simulink model "Observador_controlador"  (R2015a)
settings: Solver=ode45  SolverMode=SingleTasking  StartTime=0.0  StopTime=10.0  RelTol=1e-3
undefined symbols (not defined in the file): Ts
settings Model: CovModelRefEnable=off  Creator=n221  LastModifiedBy=ARTURO
settings DataIOCC: SignalLoggingSaveFormat=ModelDataLogs
settings OptimizationCC: BlockReduction=off  BooleanDataType=off  ExpressionDepthLimit=2147483647
settings DebuggingCC: SaveWithParameterizedLinksMsg=none  UnderspecifiedInitializationDetection=Classic  MergeDetectMultiDrivingBlocksExec=none  SignalResolutionControl=TryResolveAllWithWarning  MultiTaskDSMMsg=warning  MultiTaskCondExecSysMsg=none  StateNameClashWarn=warning
settings HardwareCC: TargetUnknown=on

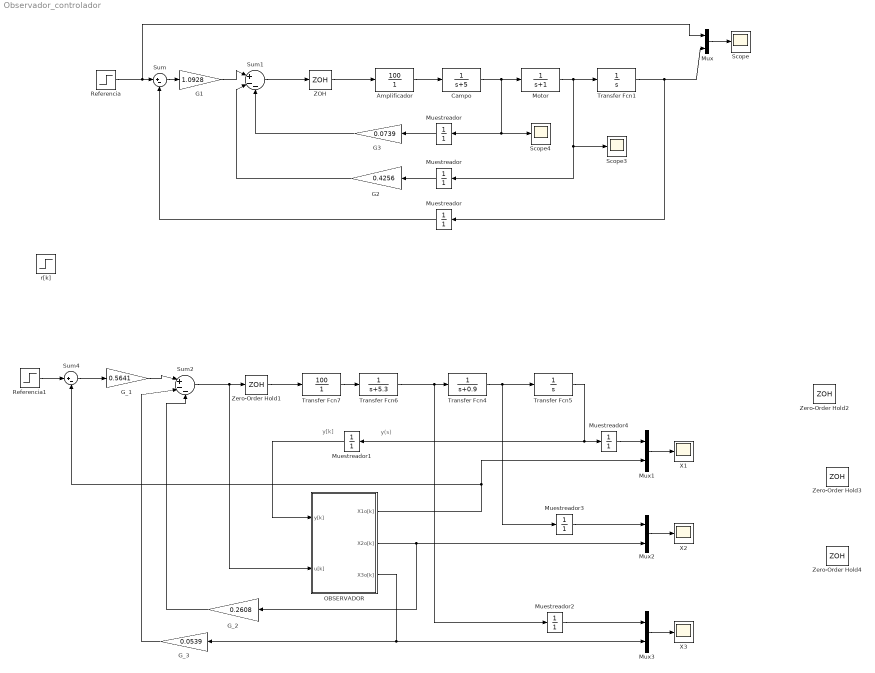
== system Observador_controlador ==
  note: y[k]
  note: y(s)
   Muestreador{,1..4} (5 alike) : DiscreteTransferFcn  Denominator=[1]  SampleTime=Ts
  Amplificador : TransferFcn  Numerator=[100]  Denominator=[1]
  Campo : TransferFcn  Denominator=[1 5]
  G1 : Gain  Gain=1.0928
  G2 : Gain  Gain=0.4256
  G3 : Gain  Gain=0.0739
  G_1 : Gain  Gain=0.5641
  G_2 : Gain  Gain=0.2608
  G_3 : Gain  Gain=0.0539
  Motor : TransferFcn  Denominator=[1 1]
  Muestreador : DiscreteTransferFcn  Denominator=[1]  SampleTime=Ts
  "Muestreador " : DiscreteTransferFcn  Denominator=[1]  SampleTime=Ts
  Mux{,1..3} (4 alike) : Mux  Inputs=2
  OBSERVADOR : Subsystem
  Referencia : Step  Time=0  SampleTime=Ts
  Referencia1 : Step  Time=0  SampleTime=Ts
  Scope : Scope
      settings: YMin=-0.13042  YMax=1.1738  SaveName=input_output
  Scope3 : Scope
      settings: YMin=-0.13042  YMax=1.1738  SaveName=input_output3
  Scope4 : Scope
      settings: YMin=-0.13042  YMax=1.1738  SaveName=input_output4
  Sum : Sum  Inputs=|+-
  Sum1 : Sum  Inputs=|+--
  Sum2 : Sum  Inputs=|+--
  Sum4 : Sum  Inputs=|+-
  Transfer Fcn1 : TransferFcn  Denominator=[1 0]
  Transfer Fcn4 : TransferFcn  Denominator=[1 0.9]
  Transfer Fcn5 : TransferFcn  Denominator=[1 0]
  Transfer Fcn6 : TransferFcn  Denominator=[1 5.3]
  Transfer Fcn7 : TransferFcn  Numerator=[100]  Denominator=[1]
  X1 : Scope
      settings: YMin=-0.13042  YMax=1.1738  SaveName=X1O
  X2 : Scope
      settings: YMin=-0.13042  YMax=1.1738  SaveName=X2O
  X3 : Scope
      settings: YMin=-0.13042  YMax=1.1738  SaveName=X3O
  ZOH : ZeroOrderHold  SampleTime=Ts
  Zero-Order Hold{1..4} (4 alike) : ZeroOrderHold  SampleTime=Ts
  r[k] : Step  Time=0  SampleTime=Ts
  wires:
  Motor/1 -> "Muestreador "/1, Scope3/1, Transfer Fcn1/1
  Campo/1 -> Muestreador/1, Scope4/1, Motor/1
  Amplificador/1 -> Campo/1
  ZOH/1 -> Amplificador/1
  Sum/1 -> G1/1
  Referencia/1 -> Sum/1, Mux/1
  G2/1 -> Sum1/2
  G1/1 -> Sum1/1
  Muestreador/1 -> G3/1
  "Muestreador "/1 -> G2/1
  Mux/1 -> Scope/1
  Transfer Fcn6/1 -> " Muestreador2"/1, Transfer Fcn4/1
  Transfer Fcn7/1 -> Transfer Fcn6/1
  Zero-Order Hold1/1 -> Transfer Fcn7/1
  " Muestreador"/1 -> Sum/2
  G3/1 -> Sum1/3
  Sum2/1 -> OBSERVADOR/2(u[k]), Zero-Order Hold1/1
  Referencia1/1 -> Sum4/1
  Sum4/1 -> G_1/1
  G_1/1 -> Sum2/1
  G_2/1 -> Sum2/3
  G_3/1 -> Sum2/2
  Mux1/1 -> X1/1
  OBSERVADOR/1(X1o[k]) -> Sum4/2, Mux1/2
  Transfer Fcn4/1 -> " Muestreador3"/1, Transfer Fcn5/1
  Mux2/1 -> X2/1
  OBSERVADOR/2(X2o[k]) -> Mux2/2, G_2/1
  Mux3/1 -> X3/1
  " Muestreador1"/1 -> OBSERVADOR/1(y[k])
  " Muestreador2"/1 -> Mux3/1
  " Muestreador3"/1 -> Mux2/1
  Transfer Fcn1/1 -> " Muestreador"/1, Mux/2
  Transfer Fcn5/1 -> " Muestreador1"/1, " Muestreador4"/1
  " Muestreador4"/1 -> Mux1/1
  Sum1/1 -> ZOH/1
  OBSERVADOR/3(X3o[k]) -> Mux3/2, G_3/1

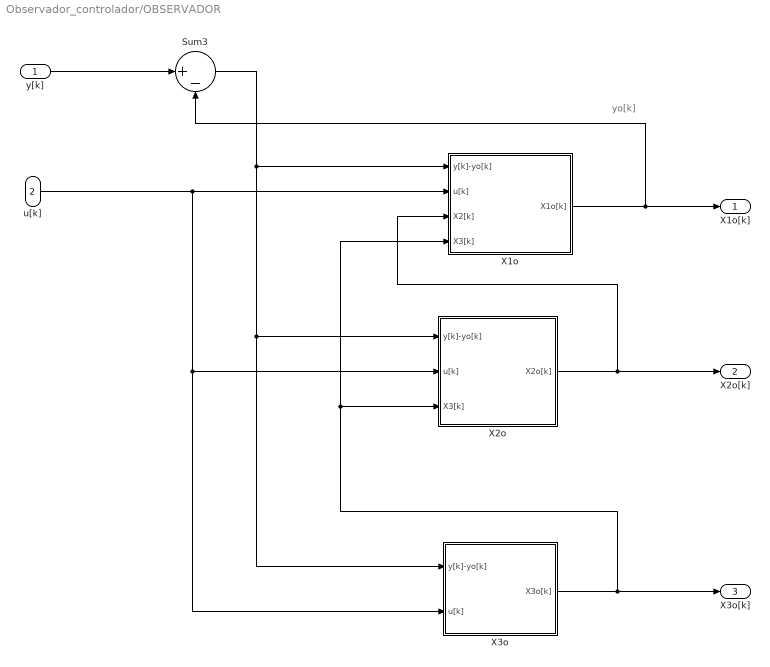
== system Observador_controlador/OBSERVADOR ==
  note: yo[k]
  y[k] : Inport
  u[k] : Inport  Port=2
  Sum3 : Sum  Inputs=|+-
  X1o : Subsystem
  X2o : Subsystem
  X3o : Subsystem
  X1o[k] : Outport
  X2o[k] : Outport  Port=2
  X3o[k] : Outport  Port=3
  wires:
  y[k]/1 -> Sum3/1
  Sum3/1 -> X3o/1(y[k]-yo[k]), X2o/1(y[k]-yo[k]), X1o/1(y[k]-yo[k])
  X2o/1(X2o[k]) -> X2o[k]/1, X1o/3(X2[k])
  u[k]/1 -> X3o/2(u[k]), X2o/2(u[k]), X1o/2(u[k])
  X3o/1(X3o[k]) -> X3o[k]/1, X2o/3(X3[k]), X1o/4(X3[k])
  X1o/1(X1o[k]) -> X1o[k]/1, Sum3/2

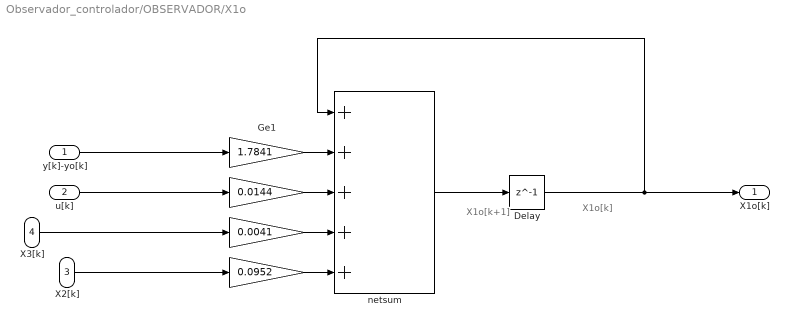
== system Observador_controlador/OBSERVADOR/X1o ==
  note: X1o[k]
  note: X1o[k+1]
  y[k]-yo[k] : Inport
  u[k] : Inport  Port=2
  X2[k] : Inport  Port=3
  X3[k] : Inport  Port=4
  " " : Gain  Gain=0.0144
  "   " : Gain  Gain=0.0952
  "    " : Gain  Gain=0.0041
  Delay : Delay  DelayLength=1  InitialCondition=0
  Ge1 : Gain  Gain=1.7841
  netsum : Sum  Inputs=5  SaturateOnIntegerOverflow=on  InputSameDT=on  OutDataTypeStr=Inherit: Same as first input
  X1o[k] : Outport
  wires:
  " "/1 -> netsum/3
  "    "/1 -> netsum/4
  "   "/1 -> netsum/5
  netsum/1 -> Delay/1
  Ge1/1 -> netsum/2
  Delay/1 -> netsum/1, X1o[k]/1
  X3[k]/1 -> "    "/1
  u[k]/1 -> " "/1
  X2[k]/1 -> "   "/1
  y[k]-yo[k]/1 -> Ge1/1

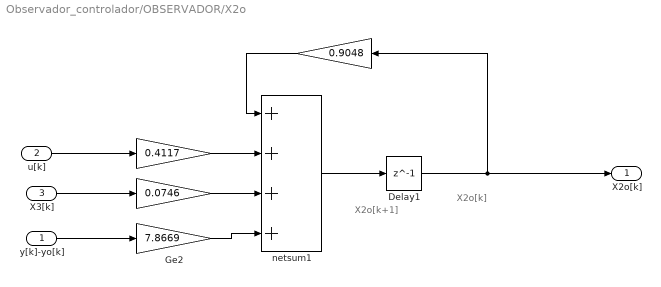
== system Observador_controlador/OBSERVADOR/X2o ==
  note: X2o[k]
  note: X2o[k+1]
  y[k]-yo[k] : Inport
  u[k] : Inport  Port=2
  X3[k] : Inport  Port=3
  " " : Gain  Gain=0.4117
  " " : Gain  Gain=0.9048
  "     " : Gain  Gain=0.0746
  Delay1 : Delay  DelayLength=1  InitialCondition=0
  Ge2 : Gain  Gain=7.8669
  netsum1 : Sum  Inputs=4  SaturateOnIntegerOverflow=on  InputSameDT=on  OutDataTypeStr=Inherit: Same as first input
  X2o[k] : Outport
  wires:
  X3[k]/1 -> "     "/1
  Delay1/1 -> " "/1, X2o[k]/1
  u[k]/1 -> " "/1
  " "/1 -> netsum1/2
  " "/1 -> netsum1/1
  netsum1/1 -> Delay1/1
  Ge2/1 -> netsum1/4
  "     "/1 -> netsum1/3
  y[k]-yo[k]/1 -> Ge2/1

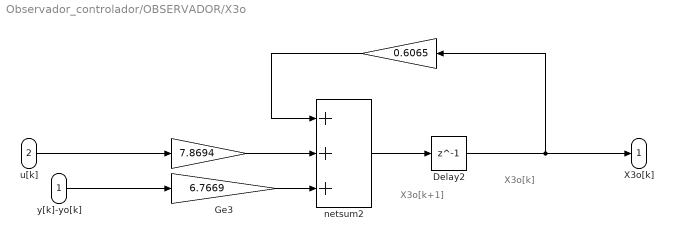
== system Observador_controlador/OBSERVADOR/X3o ==
  note: X3o[k]
  note: X3o[k+1]
  y[k]-yo[k] : Inport
  u[k] : Inport  Port=2
  " " : Gain  Gain=7.8694
  " " : Gain  Gain=0.6065
  Delay2 : Delay  DelayLength=1  InitialCondition=0
  Ge3 : Gain  Gain=6.7669
  netsum2 : Sum  Inputs=3  SaturateOnIntegerOverflow=on  InputSameDT=on  OutDataTypeStr=Inherit: Same as first input
  X3o[k] : Outport
  wires:
  netsum2/1 -> Delay2/1
  " "/1 -> netsum2/1
  Ge3/1 -> netsum2/3
  " "/1 -> netsum2/2
  u[k]/1 -> " "/1
  y[k]-yo[k]/1 -> Ge3/1
  Delay2/1 -> X3o[k]/1, " "/1
